simulink model "imu"  (Simulink 7.5)
settings: Solver=ode45  StartTime=0.0  StopTime=10.0  RelTol=1e-3
libraries: aerolibutil x1, aerolibtransform2 x1
settings Model: Creator=auvt  LastModifiedBy=micah

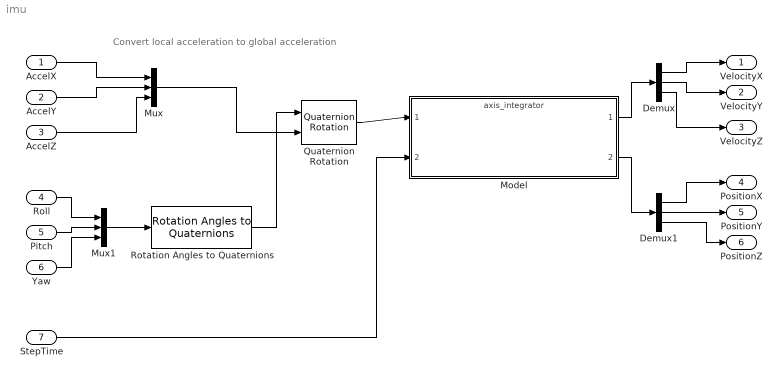
== system imu ==
  note: Convert local acceleration to global acceleration
  AccelX : Inport  OutDataType=fixdt(1, 16)  OutScaling=2^0
  AccelY : Inport  Port=2  OutDataType=fixdt(1, 16)  OutScaling=2^0
  AccelZ : Inport  Port=3  OutDataType=fixdt(1, 16)  OutScaling=2^0
  Roll : Inport  Port=4  OutDataType=fixdt(1, 16)  OutScaling=2^0
  Pitch : Inport  Port=5  OutDataType=fixdt(1, 16)  OutScaling=2^0
  Yaw : Inport  Port=6  OutDataType=fixdt(1, 16)  OutScaling=2^0
  StepTime : Inport  Port=7  OutDataType=fixdt(1, 16)  OutScaling=2^0
  Demux : Demux  Outputs=3
  Demux1 : Demux  Outputs=3
  Model : ModelReference  ModelNameDialog=axis_integrator  SimulationMode=Accelerator  ModelReferenceVersion=1.3  CopyOfModelName=axis_integrator
  Mux : Mux  Inputs=3
  Mux1 : Mux  Inputs=3
  Quaternion Rotation : aerolibutil/Quaternion Rotation  SystemSampleTime=-1
  Rotation Angles to Quaternions : aerolibtransform2/Rotation Angles to Quaternions  SystemSampleTime=-1  rotationOrder=ZYX
  VelocityX : Outport  OutDataType=fixdt(1, 16)  OutScaling=2^0
  VelocityY : Outport  Port=2  OutDataType=fixdt(1, 16)  OutScaling=2^0
  VelocityZ : Outport  Port=3  OutDataType=fixdt(1, 16)  OutScaling=2^0
  PositionX : Outport  Port=4  OutDataType=fixdt(1, 16)  OutScaling=2^0
  PositionY : Outport  Port=5  OutDataType=fixdt(1, 16)  OutScaling=2^0
  PositionZ : Outport  Port=6  OutDataType=fixdt(1, 16)  OutScaling=2^0
  wires:
  AccelX/1 -> Mux/1
  AccelY/1 -> Mux/2
  AccelZ/1 -> Mux/3
  Roll/1 -> Mux1/1
  Pitch/1 -> Mux1/2
  Yaw/1 -> Mux1/3
  Mux1/1 -> Rotation Angles to Quaternions/1
  Rotation Angles to Quaternions/1 -> Quaternion Rotation/1
  Mux/1 -> Quaternion Rotation/2
  Quaternion Rotation/1 -> Model/1
  StepTime/1 -> Model/2
  Model/1 -> Demux/1
  Model/2 -> Demux1/1
  Demux/1 -> VelocityX/1
  Demux/2 -> VelocityY/1
  Demux/3 -> VelocityZ/1
  Demux1/1 -> PositionX/1
  Demux1/2 -> PositionY/1
  Demux1/3 -> PositionZ/1
